simulink subsystem "EnergyElectric"  (R2024b)
settings: Solver=VariableStepAuto  StartTime=0.0  StopTime=10.0  RelTol=1e-3
settings Model: Creator=jjha  LastModifiedBy=saprasad
settings RTWCC: GPUComputeCapability=3.5

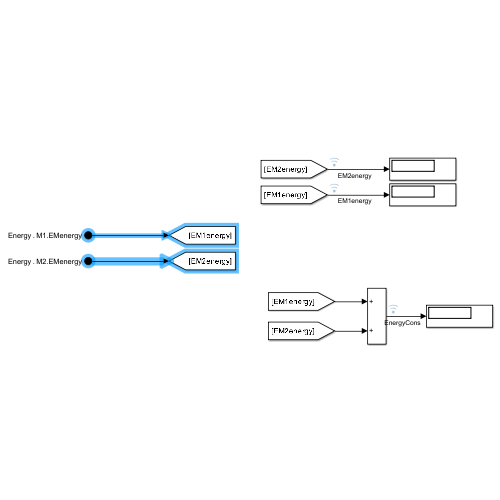
[thumbnail: Simulink's stored preview of the top-level diagram]
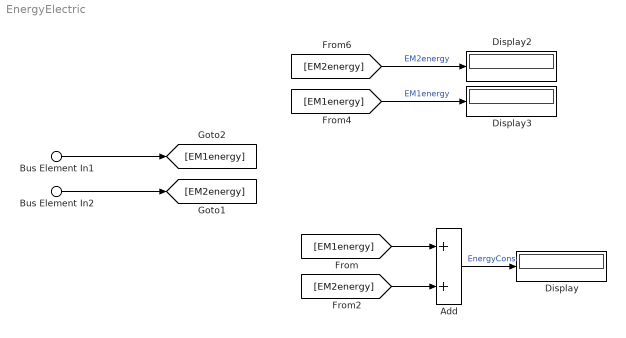
== system EnergyElectric ==
  Bus Element In1 : Inport  PortName=Energy  Element=M1.EMenergy
  Bus Element In2 : Inport  PortName=Energy  Element=M2.EMenergy
  Add : Sum
  Display : Display
  Display2 : Display
  Display3 : Display
  wires:
  [EM2energy] -> Add/2
  [EM1energy] -> Add/1
  Add/1 -> Display/1  "EnergyCons"
  [EM2energy] -> Display2/1  "EM2energy"
  [EM1energy] -> Display3/1  "EM1energy"
  Bus Element In1/1 -> [EM1energy]
  Bus Element In2/1 -> [EM2energy]
